simulink model "condenser"  (R2017b)
settings: Solver=VariableStepAuto  StartTime=0.0  StopTime=10.0  RelTol=1e-3
settings Model: Creator=Bailey Brookes  LastModifiedBy=Bailey Brookes

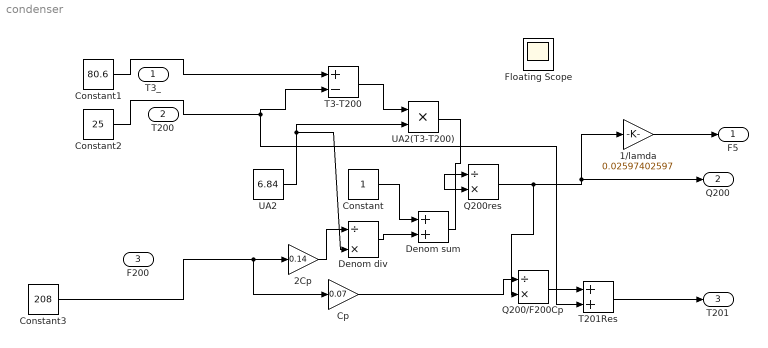
== system condenser ==
  T3_ : Inport
  T200 : Inport  Port=2
  F200 : Inport  Port=3
  1/lamda : Gain  Gain=0.02597402597
  2Cp : Gain  Gain=0.14
  Constant : Constant
  Constant1 : Constant  Value=80.6
  Constant2 : Constant  Value=25
  Constant3 : Constant  Value=208
  Cp : Gain  Gain=0.07
  Denom div : Product  Inputs=/*
  Denom sum : Sum
  Floating Scope : Scope
      settings: Floating=on
  Q200/F200Cp : Product  Inputs=/*
  Q200res : Product  Inputs=/*
  T201Res : Sum
  T3-T200 : Sum  Inputs=+-
  UA2 : Constant  Value=6.84
  UA2(T3-T200) : Product
  F5 : Outport
  Q200 : Outport  Port=2
  T201 : Outport  Port=3
  wires:
  UA2/1 -> Denom div/2, UA2(T3-T200)/2
  Cp/1 -> Q200/F200Cp/1
  Constant3/1 -> 2Cp/1, Cp/1
  Denom div/1 -> Denom sum/2
  Constant/1 -> Denom sum/1
  T3-T200/1 -> UA2(T3-T200)/1
  T201Res/1 -> T201/1
  Constant1/1 -> T3-T200/1
  Q200/F200Cp/1 -> T201Res/1
  Constant2/1 -> T201Res/2, T3-T200/2
  Q200res/1 -> Q200/F200Cp/2, 1/lamda/1, Q200/1
  Denom sum/1 -> Q200res/1
  UA2(T3-T200)/1 -> Q200res/2
  1/lamda/1 -> F5/1
  2Cp/1 -> Denom div/1
